simulink model "High_Gain_control_1"  (R2018b)
settings: Solver=VariableStepAuto  StartTime=0.0  StopTime=2  RelTol=1e-3
InitFcn:
  | %参数初始化
  | a = 0.7;
settings Model: Creator=Think  LastModifiedBy=Think

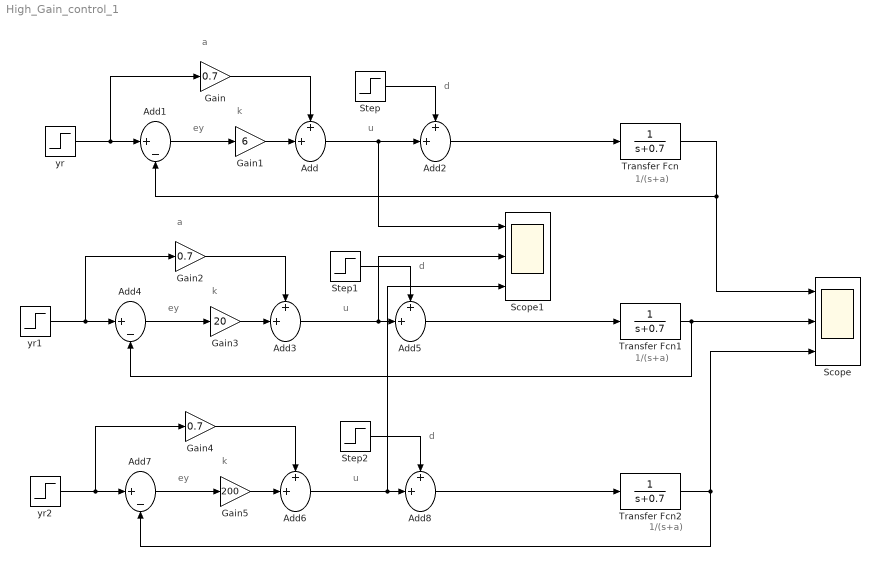
== system High_Gain_control_1 ==
  note: k
  note: ey
  note: a
  note: d
  note: u
  note: 1/(s+a)
  note: k
  note: ey
  note: a
  note: d
  note: u
  note: 1/(s+a)
  note: k
  note: ey
  note: d
  note: u
  note: 1/(s+a)
  Add{,2..3,5..6,8} (6 alike) : Sum  Inputs=++|
  Add1 : Sum  Inputs=|+-
  Add4 : Sum  Inputs=|+-
  Add7 : Sum  Inputs=|+-
  Gain : Gain  Gain=0.7
  Gain1 : Gain  Gain=6
  Gain2 : Gain  Gain=0.7
  Gain3 : Gain  Gain=20
  Gain4 : Gain  Gain=0.7
  Gain5 : Gain  Gain=200
  Scope : Scope  NumInputPorts=3
  Scope1 : Scope  NumInputPorts=3
  Step : Step  After=2  SampleTime=0
  Step1 : Step  After=2  SampleTime=0
  Step2 : Step  After=2  SampleTime=0
  Transfer Fcn : TransferFcn  Denominator=[1 0.7]
  Transfer Fcn1 : TransferFcn  Denominator=[1 0.7]
  Transfer Fcn2 : TransferFcn  Denominator=[1 0.7]
  yr : Step  Time=0  After=2  SampleTime=0
  yr1 : Step  Time=0  After=2  SampleTime=0
  yr2 : Step  Time=0  After=2  SampleTime=0
  wires:
  Gain/1 -> Add/1
  Gain1/1 -> Add/2
  Add1/1 -> Gain1/1
  Add/1 -> Scope1/1, Add2/2
  Step/1 -> Add2/1
  Add2/1 -> Transfer Fcn/1
  yr/1 -> Gain/1, Add1/1
  Transfer Fcn/1 -> Add1/2, Scope/1
  Transfer Fcn1/1 -> Scope/2, Add4/2
  yr1/1 -> Add4/1, Gain2/1
  Add5/1 -> Transfer Fcn1/1
  Step1/1 -> Add5/1
  Add3/1 -> Scope1/2, Add5/2
  Add4/1 -> Gain3/1
  Gain3/1 -> Add3/2
  Gain2/1 -> Add3/1
  Gain4/1 -> Add6/1
  Gain5/1 -> Add6/2
  Add7/1 -> Gain5/1
  Add6/1 -> Scope1/3, Add8/2
  Step2/1 -> Add8/1
  Add8/1 -> Transfer Fcn2/1
  yr2/1 -> Gain4/1, Add7/1
  Transfer Fcn2/1 -> Scope/3, Add7/2
